simulink model "Unattended Object Detection"  (R2013b)
settings: Solver=ode45  StartTime=0.0  StopTime=inf  RelTol=1e-3
undefined symbols (not defined in the file): Rec, SDTV, strel
libraries: visionconversions x2, visionstatistics x1, visiontextngfix x1, dspvision x1, visionanalysis x1, simulink x1, visionmorphops x1
settings Model: Creator=Ajay  LastModifiedBy=Ajay

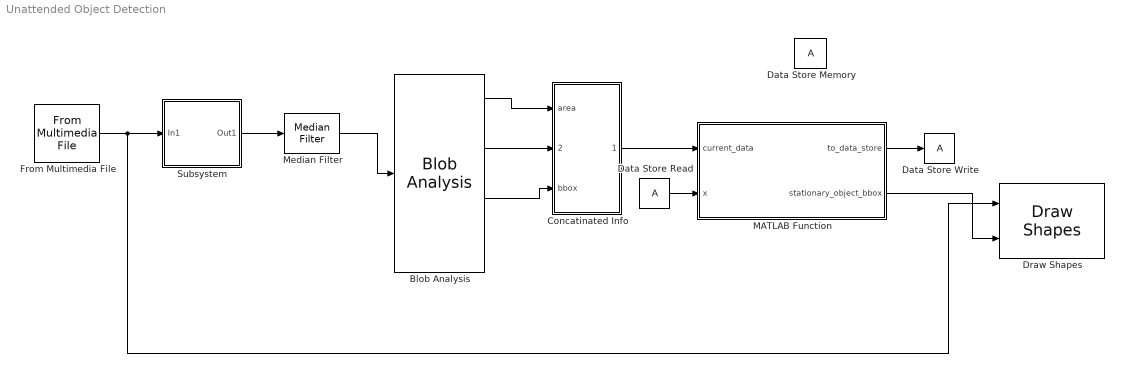
== system Unattended Object Detection ==
  Blob Analysis : visionstatistics/Blob Analysis  Tag=vipblks_row_conv  area=on  centroid=on  bBox=on  majorAxis=off  minorAxis=off  angle=off  eccentricity=off  equivDiameterSq=off  extent=off  perimeter=off  maxBlobs=50  warnIfNumBlobsExceeded=off  isCount=off  useMinArea=on  minArea=200  useMaxArea=on  maxArea=10000  excludeBorderBlob=on  outDT=single  isOutVarDim=off  isFill=on  fillValues=-1  conn=4  isLabel=on  outputMode=Binary point scaling  outputWordLength=32  outputFracLength=16  firstCoeffMode=Binary point scaling  firstCoeffWordLength=16  firstCoeffFracLength=14  secondCoeffMode=Binary point scaling  secondCoeffWordLength=32  secondCoeffFracLength=16  accumMode=Binary point scaling  accumWordLength=32  accumFracLength=0  prodOutputMode=Binary point scaling  prodOutputWordLength=32  prodOutputFracLength=16  roundingMode=Floor  overflowMode=off
  Concatinated Info : MATLAB Function  TreatAsAtomicUnit=on
  Data Store Memory : DataStoreMemory  ReadBeforeWriteMsg=warning  WriteAfterWriteMsg=warning  WriteAfterReadMsg=warning  InitialValue=[0]
  Data Store Read : DataStoreRead
  Data Store Write : DataStoreWrite
  Draw Shapes : visiontextngfix/Draw Shapes  shape=Rectangles  fill=off  fillClrSource=Specify via dialog  display=User-specified value  intensity=200  color=[255 0 0]  opacity=0.6  viewport=Entire image  antialiasing=off  inType=Obsolete  imagePorts=One multidimensional signal  prodOutputMode=Binary point scaling  prodOutputWordLength=32  prodOutputFracLength=14  memoryMode=Specify word length  memoryWordLength=16  memoryFracLength=15  roundingMode=Floor  overflowMode=off
  From Multimedia File : dspvision/From Multimedia File  inputFilename=C:\Users\Ajay\Documents\Adobe\Premiere Pro\9.0\Sequence 01.avi  loop=on  numPlays=inf  outputStreams=Video only  videoDataType=single  audioDataType=int16  inheritSampleTime=on  userDefinedSampleTime=1/30  noAudioOutput=off  isIntensityVideo=off  fourcc=RGB  colorVideoFormat=One multidimensional signal  outputEOF=off  dataOrg=Column-major  audioFrameSize=1024  computeAudioFrameSize=off  outSamplingMode=Sample based
  MATLAB Function : MATLAB Function  TreatAsAtomicUnit=on
  Median Filter : visionanalysis/Median Filter  nghbood=[10 10]  outSize=Same as input port I  padType=Constant  padSrc=Specify via dialog  padVal=0  roundingMode=Floor  overflowMode=off
  Subsystem : Subsystem
  wires:
  From Multimedia File/1 -> Draw Shapes/1, Subsystem/1(In1)
  Subsystem/1(Out1) -> Median Filter/1
  Median Filter/1 -> Blob Analysis/1
  Blob Analysis/3 -> Concatinated Info/3(bbox)
  Blob Analysis/2 -> Concatinated Info/2(centroid)
  Blob Analysis/1 -> Concatinated Info/1(area)
  MATLAB Function/1(to_data_store) -> Data Store Write/1
  Data Store Read/1 -> MATLAB Function/2(x)
  MATLAB Function/2(stationary_object_bbox) -> Draw Shapes/2
  Concatinated Info/1(current_data) -> MATLAB Function/1(current_data)

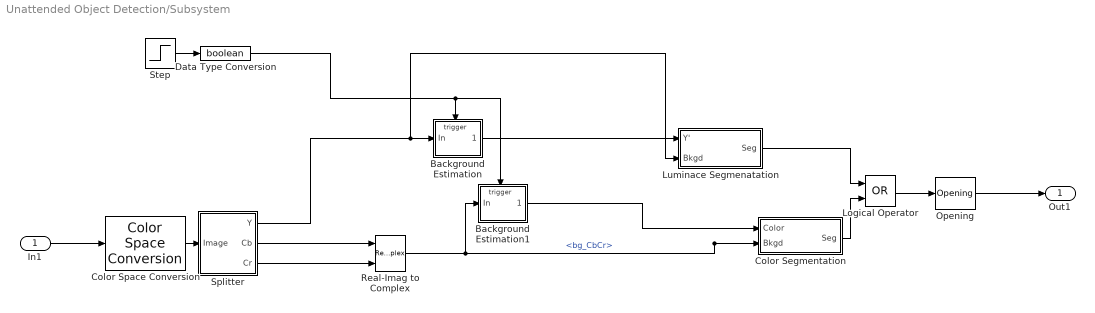
== system Unattended Object Detection/Subsystem ==
  In1 : Inport
  Background Estimation : Subsystem  TreatAsAtomicUnit=on  mask{initCond=0}
      mask prompts: initCond "Initial Condition"
  Background Estimation1 : Subsystem  TreatAsAtomicUnit=on  mask{initCond=0}
      mask prompts: initCond "Initial Condition"
  Color Segmentation : Subsystem
      settings: RTWMemSecFuncInitTerm=Default  RTWMemSecFuncExecute=Default  RTWMemSecDataConstants=Default  RTWMemSecDataInternal=Default  RTWMemSecDataParameters=Default
  Color Space Conversion : visionconversions/Color Space  Conversion  conversion=Obsolete  conversionActive=R'G'B' to Y'CbCr  wp_str=D65  rec=Rec. 601 (SDTV)  sys=1125/60/2:1  imagePorts=One multidimensional signal
  Data Type Conversion : DataTypeConversion  OutDataTypeStr=boolean
  Logical Operator : Logic  Operator=OR  AllPortsSameDT=off  OutDataTypeStr=boolean
  Luminace Segmenatation : Subsystem
      settings: RTWMemSecFuncInitTerm=Default  RTWMemSecFuncExecute=Default  RTWMemSecDataConstants=Default  RTWMemSecDataInternal=Default  RTWMemSecDataParameters=Default
  Opening : visionmorphops/Opening  nhoodsrc=Specify via dialog  strel=strel('square',3)
  Real-Imag to Complex : RealImagToComplex
  Splitter : Subsystem
  Step : Step  Time=eps
  Out1 : Outport
  wires:
  Background Estimation/1(" ") -> Luminace Segmenatation/1(Y')
  Splitter/1(Y) -> Luminace Segmenatation/2(Bkgd), Background Estimation/1(In)
  Background Estimation1/1(" ") -> Color Segmentation/1(Color)
  Real-Imag to Complex/1 -> Color Segmentation/2(Bkgd), Background Estimation1/1(In)  "<bg_CbCr>"
  Luminace Segmenatation/1(Seg) -> Logical Operator/1
  Color Segmentation/1(Seg) -> Logical Operator/2
  Logical Operator/1 -> Opening/1
  Splitter/3(Cr) -> Real-Imag to Complex/2
  Splitter/2(Cb) -> Real-Imag to Complex/1
  Data Type Conversion/1 -> Background Estimation/Trigger, Background Estimation1/Trigger
  Step/1 -> Data Type Conversion/1
  In1/1 -> Color Space Conversion/1
  Color Space Conversion/1 -> Splitter/1(Image)
  Opening/1 -> Out1/1

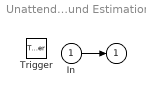
== system Unattended Object Detection/Subsystem/Background Estimation ==
  In : Inport
  Trigger : TriggerPort  ZeroCross=off
  " " : Outport  InitialOutput=initCond
  wires:
  In/1 -> " "/1

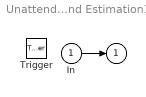
== system Unattended Object Detection/Subsystem/Background Estimation1 ==
  In : Inport
  Trigger : TriggerPort  ZeroCross=off
  " " : Outport  InitialOutput=initCond
  wires:
  In/1 -> " "/1

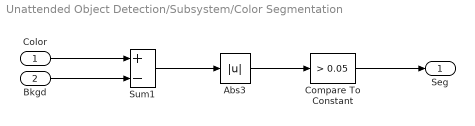
== system Unattended Object Detection/Subsystem/Color Segmentation ==
  Color : Inport
  Bkgd : Inport  Port=2
  Abs3 : Abs  SaturateOnIntegerOverflow=on
  Compare To Constant : simulink/Logic and Bit Operations/Compare To Constant  relop=>  const=0.05  OutDataTypeStr=boolean  ZeroCross=off
  Sum1 : Sum  Inputs=+-  SaturateOnIntegerOverflow=on  InputSameDT=on  OutDataTypeStr=Inherit: Same as first input
  Seg : Outport
  wires:
  Bkgd/1 -> Sum1/2
  Color/1 -> Sum1/1
  Sum1/1 -> Abs3/1
  Compare To Constant/1 -> Seg/1
  Abs3/1 -> Compare To Constant/1

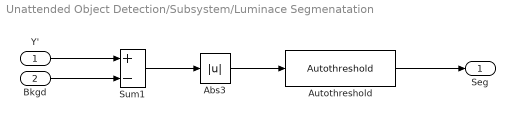
== system Unattended Object Detection/Subsystem/Luminace Segmenatation ==
  Y' : Inport
  Bkgd : Inport  Port=2
  Abs3 : Abs  SaturateOnIntegerOverflow=on
  Autothreshold : visionconversions/Autothreshold  operator=>  threshOut=off  effMetricOut=off  userDefinedRange=off  umin=0  umax=100  outOfRngOpt=Warn and saturate  scaleThreshold=on  scaleFactor=1.3  P1Mode=Specify word length  P1WordLength=32  P1FracLength=30  P2Mode=Specify word length  P2WordLength=32  P2FracLength=22  P3Mode=Specify word length  P3WordLength=32  P3FracLength=14  P4Mode=Binary point scaling  P4WordLength=32  P4FracLength=15  Q1Mode=Specify word length  Q1WordLength=32  Q1FracLength=16  EMMode=Specify word length  EMWordLength=16  EMFracLength=14  roundingMode=Floor  overflowMode=off
  Sum1 : Sum  Inputs=+-  SaturateOnIntegerOverflow=on  InputSameDT=on  OutDataTypeStr=Inherit: Same as first input
  Seg : Outport
  wires:
  Abs3/1 -> Autothreshold/1
  Autothreshold/1 -> Seg/1
  Sum1/1 -> Abs3/1
  Y'/1 -> Sum1/1
  Bkgd/1 -> Sum1/2

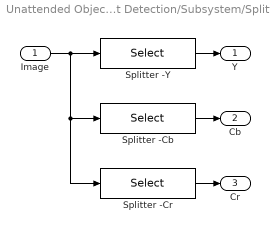
== system Unattended Object Detection/Subsystem/Splitter ==
  Image : Inport
  Splitter -Cb : Selector  NumberOfDimensions=3  IndexOptions=Select all,Select all,Index vector (dialog)  Indices=[],[],[2]  OutputSizes=1
  Splitter -Cr : Selector  NumberOfDimensions=3  IndexOptions=Select all,Select all,Index vector (dialog)  Indices=[],[],[3]  OutputSizes=1
  Splitter -Y : Selector  NumberOfDimensions=3  IndexOptions=Select all,Select all,Index vector (dialog)  Indices=[],[],[1]  OutputSizes=1
  Y : Outport
  Cb : Outport  Port=2
  Cr : Outport  Port=3
  wires:
  Image/1 -> Splitter -Cr/1, Splitter -Cb/1, Splitter -Y/1
  Splitter -Y/1 -> Y/1
  Splitter -Cb/1 -> Cb/1
  Splitter -Cr/1 -> Cr/1

== matlab function Unattended Object Detection/MATLAB Function ==
  data: current_data input; to_data_store output; x input; stationary_object_bbox output
function [to_data_store,stationary_object_bbox]= fcn(current_data,x)
coder.extrinsic('clear')
stationary_threshold=500;
pixel_error_factor =10;
area_error_factor=30;
d=[]
dim=size(x)
if(dim(1)==1&&dim(2)==1)
   
    d=[0 0 0 0 0 0 0 0 0 0 ];
else
    d=x;
end
%{
d=d(:,8)<-10; % Remeoving rows that have count less than 10




d(:,10)=0;     % Flag =0




for i=1:length(current_data)
    x=current_data(i,1);
    y=current_data(i,2);
    area=d(i,3);
    t=0;
    for j=1:length(d)
        if((d(j,1)-pixel_error_factor<x && d(j,1)+pixel_error_factor>x) && (d(j,2)-pixel_error_factor<y && d(j,2)+pixel_error_factor>y)&&(d(j,3)-area_error_factor<area && d(j,3)+area_error_factor<area))
            d(j,8)=d(j,8)+1;
            d(j,10)=1;
            t=t+1;
        end
        
    end
    if(t==0)
        d=[d ;current_value(i) 1 0 1];
    end
end

t=100;

for i=1:length(d)
    if(d(i,10)==0)
        d(i,8)=d(i,8)-1;
    end
end

for i=1:length(d)
    if(d(i,8)>stationary_threshold)
        d(i,9)=1;
    else
        d(i,9)=0;
        
    end
end

stationary_object_bbox=[];

for i=1:length(d)
    if(d(i,9)==1)
        stationary_object_bbox=[stationary_object_bbox; d(i,4) d(i,5) d(i,6) d(i,7) ];
        
    end
end
%}
to_data_store=d;
stationary_object_bbox=[0 0 0 0]
end

== matlab function Unattended Object Detection/Concatinated Info ==
  data: area input; current_data output; centroid input; bbox input
function current_data = fcn(area,centroid,bbox)
current_data=[centroid area bbox]
end
